simulink model "EX23"  (R2014a)
settings: Solver=ode3  StartTime=0.0  StopTime=4  FixedStep=9.76562e-4  RelTol=1e-3
settings Model: Creator=Dennis Silage  LastModifiedBy=Silage
settings DataIOCC: SignalLoggingSaveFormat=ModelDataLogs
settings OptimizationCC: ExpressionDepthLimit=2147483647  InitFltsAndDblsToZero=on
settings DebuggingCC: UnderspecifiedInitializationDetection=Classic  FcnCallInpInsideContextMsg=UseLocalSettings  StateNameClashWarn=warning  StrictBusMsg=Warning
settings GRTTargetCC: CombineOutputUpdateFcns=off  GRTInterface=on

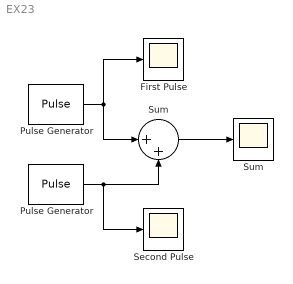
== system EX23 ==
  " Sum " : Scope
  First Pulse : Scope
      settings: SaveName=ScopeData2
  Pulse Generator : DiscretePulseGenerator  Amplitude=2  Period=4096  PulseWidth=1024  SampleTime=9.76562e-4
  "Pulse Generator " : DiscretePulseGenerator  Period=4096  PulseWidth=1024  PhaseDelay=1024  SampleTime=9.76562e-4
  Second Pulse : Scope
  Sum : Sum  Inputs=|++
  wires:
  Pulse Generator/1 -> Sum/1, First Pulse/1
  "Pulse Generator "/1 -> Sum/2, Second Pulse/1
  Sum/1 -> " Sum "/1
